simulink model "ejercicio9_EM"  (R2018a)
settings: Solver=VariableStepAuto  StartTime=0.0  StopTime=4.5  RelTol=1e-3
undefined symbols (not defined in the file): a, B1, B2, Jm, Jt, K, Ka, M, r, Ra
settings Model: Creator=carma  LastModifiedBy=carma

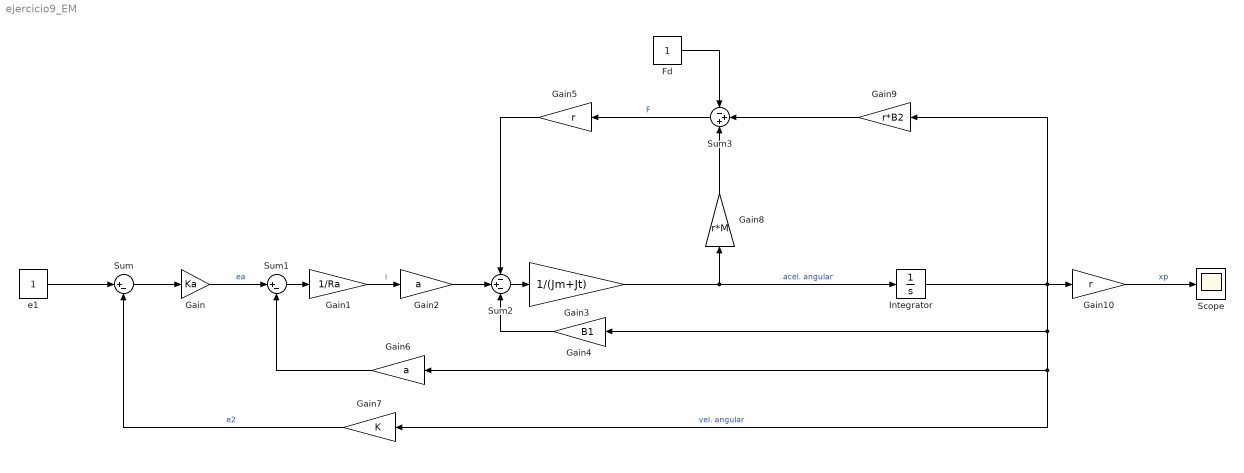
== system ejercicio9_EM ==
  Fd : Constant
  Gain : Gain  Gain=Ka
  Gain1 : Gain  Gain=1/Ra
  Gain10 : Gain  Gain=r
  Gain2 : Gain  Gain=a
  Gain3 : Gain  Gain=1/(Jm+Jt)
  Gain4 : Gain  Gain=B1
  Gain5 : Gain  Gain=r
  Gain6 : Gain  Gain=a
  Gain7 : Gain  Gain=K
  Gain8 : Gain  Gain=r*M
  Gain9 : Gain  Gain=r*B2
  Integrator : Integrator
  Scope : Scope
  Sum : Sum  Inputs=|+-
  Sum1 : Sum  Inputs=|+-
  Sum2 : Sum  Inputs=-+-
  Sum3 : Sum  Inputs=-++
  e1 : Constant
  wires:
  e1/1 -> Sum/1
  Gain7/1 -> Sum/2  "e2"
  Sum/1 -> Gain/1
  Gain/1 -> Sum1/1  "ea"
  Gain6/1 -> Sum1/2
  Sum1/1 -> Gain1/1
  Gain1/1 -> Gain2/1  "i"
  Gain2/1 -> Sum2/2
  Sum2/1 -> Gain3/1
  Gain3/1 -> Gain8/1, Integrator/1  "acel. angular"
  Integrator/1 -> Gain10/1, Gain9/1, Gain6/1, Gain7/1, Gain4/1  "vel. angular"
  Gain4/1 -> Sum2/3
  Gain5/1 -> Sum2/1
  Sum3/1 -> Gain5/1  "F"
  Gain8/1 -> Sum3/3
  Gain9/1 -> Sum3/2
  Fd/1 -> Sum3/1
  Gain10/1 -> Scope/1  "xp"
